simulink model "rlflight"  (R2022b)
settings: Solver=ode45  StartTime=0.0  StopTime=inf  RelTol=1e-3  EnableMultiTasking=on
libraries: instrumentlib x6, rllib x2
settings Model: PacingRate=10  Creator=The MathWorks, Inc.  LastModifiedBy=zzh
settings SolverCC: AlgebraicLoopSolver=TrustRegion
settings DataIOCC: LimitDataPoints=on  SaveFormat=Array  SignalLoggingName=logsOut
settings OptimizationCC: ExpressionDepthLimit=2147483647  InitFltsAndDblsToZero=on  LifeSpan=inf
settings DebuggingCC: SaveWithParameterizedLinksMsg=none  UnderspecifiedInitializationDetection=Classic  MergeDetectMultiDrivingBlocksExec=none  SignalResolutionControl=TryResolveAllWithWarning  MultiTaskDSMMsg=warning  FcnCallInpInsideContextMsg=warning  UnconnectedInputMsg=warning  UnconnectedOutputMsg=warning  UnconnectedLineMsg=warning  AllowSymbolicDim=off  StateNameClashWarn=warning  SFUnexpectedBacktrackingDiag=warning  SFNoUnconditionalDefaultTransitionDiag=warning  SFExecutionAtInitializationDiag=none  SFMachineParentedDataDiag=warning  ArithmeticOperatorsInVariantConditions=warning
settings HardwareCC: ProdBitPerPointer=32  ProdBitPerSizeT=32  ProdBitPerPtrDiffT=32  ProdLargestAtomicFloat=None  ProdIntDivRoundTo=Undefined  ProdEndianess=Unspecified  ProdWordSize=32  ProdHWDeviceType=Specified
settings ModelReferenceCC: EnableRefExpFcnMdlSchedulingChecks=on  PropagateSignalLabelsOutOfModel=off
settings SFSimCC: SimUseLocalCustomCode=off  CustomCodeUndefinedFunction=UseInterfaceOnly
settings RTWCC: RTWUseLocalCustomCode=off  DLArmComputeVersion=19.05
settings CodeAppCC: StateflowObjectComments=on
settings GRTTargetCC: TargetFcnLib=ansi_tfl_tmw.mat  TargetLangStandard=C89/C90 (ANSI)  CombineOutputUpdateFcns=off  GRTInterface=on
settings ConfigComp: CovMetricSettings=dw  CovSaveCumulativeToWorkspaceVar=on  CovSaveSingleToWorkspaceVar=on  CovExternalEMLEnable=off

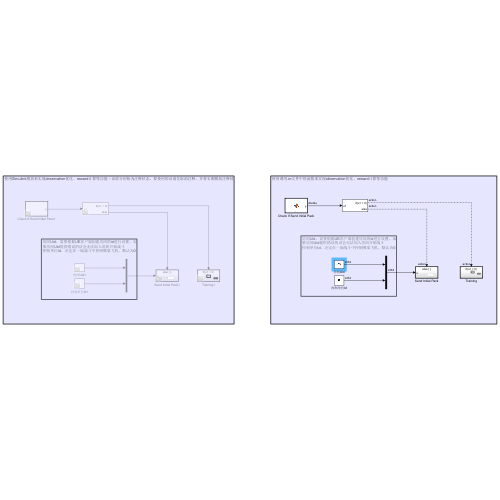
[thumbnail: Simulink's stored preview of the top-level diagram]
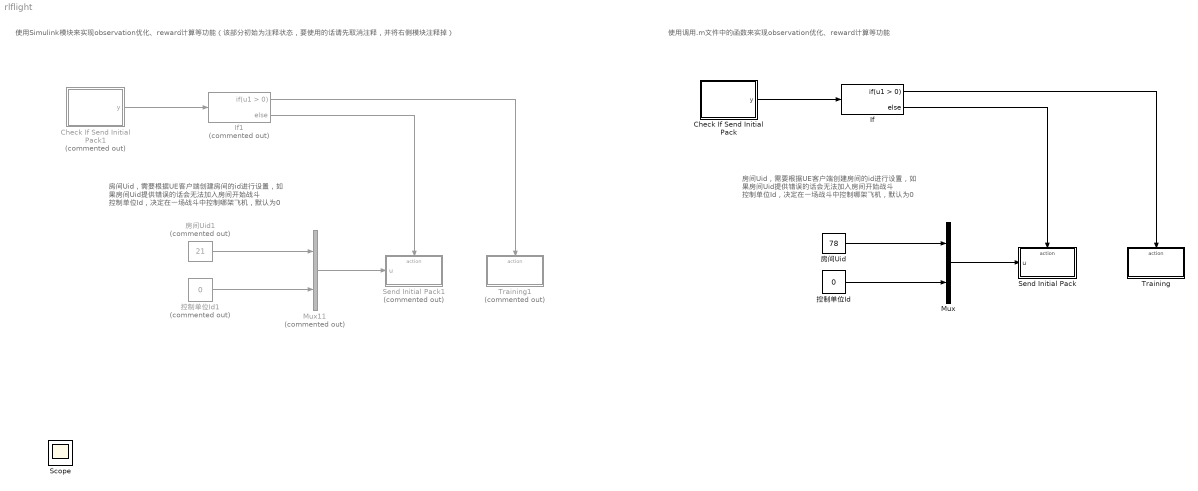
== system rlflight ==
  note: 使用调用.m文件中的函数来实现observation优化、reward计算等功能
  note: 使用Simulink模块来实现observation优化、reward计算等功能（该部分初始为注释状态，要使用的话请先取消注释，并将右侧模块注释掉）
  note: 房间Uid，需要根据UE客户端创建房间的id进行设置，如
      | 果房间Uid提供错误的话会无法加入房间开始战斗
      | 控制单位Id，决定在一场战斗中控制哪架飞机，默认为0
  note: 房间Uid，需要根据UE客户端创建房间的id进行设置，如
      | 果房间Uid提供错误的话会无法加入房间开始战斗
      | 控制单位Id，决定在一场战斗中控制哪架飞机，默认为0
  Check If Send Initial Pack : MATLAB Function  TreatAsAtomicUnit=on
  Check If Send Initial Pack1 : MATLAB Function  Commented=on  TreatAsAtomicUnit=on
  If : If
  If1 : If  Commented=on
  Mux : Mux  Inputs=2
  Mux11 : Mux  Commented=on  Inputs=2
  Send Initial Pack : Subsystem  TreatAsAtomicUnit=on
  Send Initial Pack1 : Subsystem  Commented=on  TreatAsAtomicUnit=on
  Training : Subsystem  TreatAsAtomicUnit=on
  Training1 : Subsystem  Commented=on  TreatAsAtomicUnit=on
  房间Uid : Constant  Value=78  OutDataTypeStr=int32
  房间Uid1 : Constant  Commented=on  Value=21  OutDataTypeStr=int32
  控制单位Id : Constant  Value=0  OutDataTypeStr=int32
  控制单位Id1 : Constant  Commented=on  Value=0  OutDataTypeStr=int32
  Scope : Scope
  wires:
  房间Uid/1 -> Mux/1
  控制单位Id/1 -> Mux/2
  Check If Send Initial Pack/1(y) -> If/1
  Mux/1 -> Send Initial Pack/1(u)
  If/2 -> Send Initial Pack/Action
  If/1 -> Training/Action
  控制单位Id1/1 -> Mux11/2
  Mux11/1 -> Send Initial Pack1/1(u)
  Check If Send Initial Pack1/1(y) -> If1/1
  房间Uid1/1 -> Mux11/1
  If1/2 -> Send Initial Pack1/Action
  If1/1 -> Training1/Action

== system rlflight/Send Initial Pack ==
  u : Inport
  Action Port : ActionPort  ActionPortLabel=else
  TCP发送初始信息 : instrumentlib/TCP//IP Send  Priority=1  Host=127.0.0.1  Port=8080  ByteOrder=little-endian  EnableBlockingMode=on  Timeout=5  TransferDelay=on  SimulateUsing=Interpreted execution
  wires:
  u/1 -> TCP发送初始信息/1

== system rlflight/Send Initial Pack1 ==
  u : Inport
  Action Port : ActionPort  ActionPortLabel=else
  TCP发送初始信息 : instrumentlib/TCP//IP Send  Priority=1  Host=127.0.0.1  Port=8080  ByteOrder=little-endian  EnableBlockingMode=on  Timeout=5  TransferDelay=on  SimulateUsing=Interpreted execution
  wires:
  u/1 -> TCP发送初始信息/1

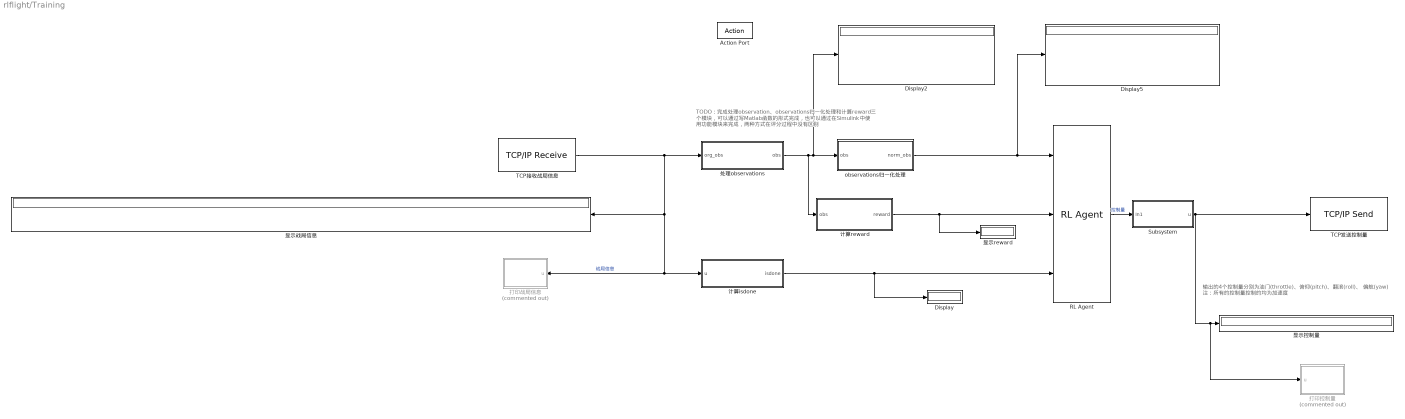
== system rlflight/Training ==
  note: 输出的4个控制量分别为油门(throttle)、俯仰(pitch)、翻滚(roll)、
      | 偏航(yaw)
      | 注：所有的控制量控制的均为加速度
  note: TODO：完成处理observation、observations归一化处理和计算reward三
      | 个模块，可以通过写Matlab函数的形式完成，也可以通过在Simulink中使
      | 用功能模块来完成，两种方式在评分过程中没有区别
  Action Port : ActionPort  ActionPortLabel=if(u1 > 0)
  Display : Display
  Display2 : Display
  Display5 : Display
  RL Agent : rllib/RL Agent  Agent=agent  ExternalActionAsInput=off  ProvideLastAction=off  ProvideCumRwd=off  TreatAsDirectFeedthrough=on  UseStrictObservationDataTypes=off
  Subsystem : Subsystem
  TCP发送控制量 : instrumentlib/TCP//IP Send  Priority=3  Host=127.0.0.1  Port=8080  ByteOrder=little-endian  EnableBlockingMode=on  Timeout=20  TransferDelay=off  SimulateUsing=Interpreted execution
  TCP接收战局信息 : instrumentlib/TCP//IP Receive  Priority=2  Host=127.0.0.1  Port=8080  DataSize=[ 1, 27 ]  DataType=double  ASCIIFormatting=%f  Terminator=LF  CustomTerminator=10  ByteOrder=little-endian  EnableBlockingMode=on  Timeout=20  SampleTime=-1  SimulateUsing=Interpreted execution
  observations归一化处理 : MATLAB Function  TreatAsAtomicUnit=on
  处理observations : MATLAB Function  TreatAsAtomicUnit=on
  打印战局信息 : MATLAB Function  Commented=on  TreatAsAtomicUnit=on
  打印控制量 : MATLAB Function  Commented=on  TreatAsAtomicUnit=on
  显示reward : Display
  显示战局信息 : Display
  显示控制量 : Display
  计算isdone : MATLAB Function  TreatAsAtomicUnit=on
  计算reward : MATLAB Function  TreatAsAtomicUnit=on
  wires:
  计算reward/1(reward) -> 显示reward/1, RL Agent/2
  计算isdone/1(isdone) -> Display/1, RL Agent/3
  TCP接收战局信息/1 -> 打印战局信息/1(u), 计算isdone/1(u), 显示战局信息/1, 处理observations/1(org_obs)  "战局信息"
  observations归一化处理/1(norm_obs) -> Display5/1, RL Agent/1
  处理observations/1(obs) -> 计算reward/1(obs), Display2/1, observations归一化处理/1(obs)
  RL Agent/1 -> Subsystem/1(In1)  "控制量"
  Subsystem/1(u) -> 打印控制量/1(u), 显示控制量/1, TCP发送控制量/1

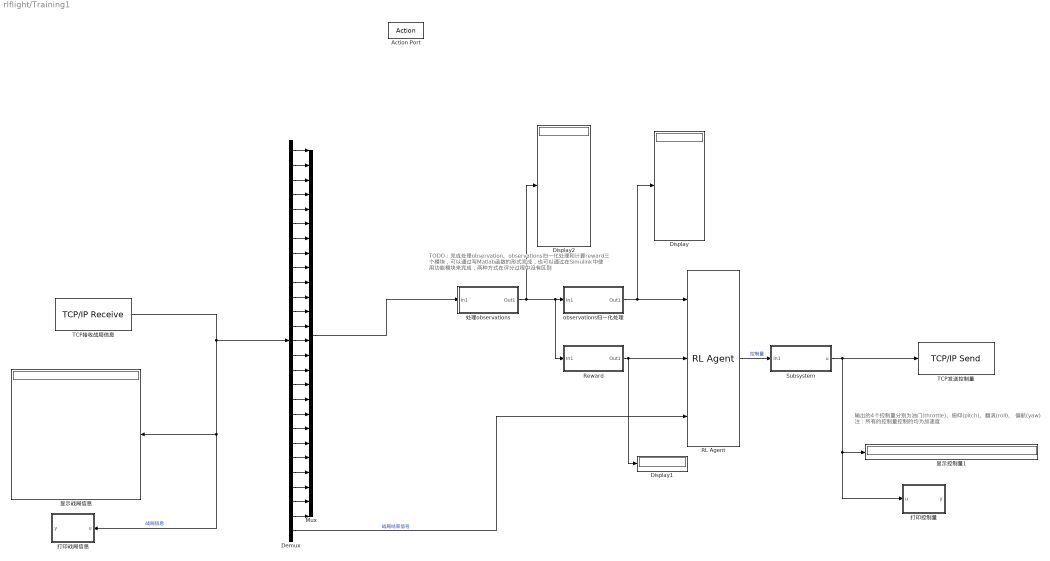
== system rlflight/Training1 ==
  note: 输出的4个控制量分别为油门(throttle)、俯仰(pitch)、翻滚(roll)、
      | 偏航(yaw)
      | 注：所有的控制量控制的均为加速度
  note: TODO：完成处理observation、observations归一化处理和计算reward三
      | 个模块，可以通过写Matlab函数的形式完成，也可以通过在Simulink中使
      | 用功能模块来完成，两种方式在评分过程中没有区别
  Action Port : ActionPort  ActionPortLabel=if(u1 > 0)
  Demux : Demux  Outputs=27
  Display : Display
  Display1 : Display
  Display2 : Display
  Mux : Mux  Inputs=26
  RL Agent : rllib/RL Agent  Agent=agent  ExternalActionAsInput=off  ProvideLastAction=off  ProvideCumRwd=off  TreatAsDirectFeedthrough=on  UseStrictObservationDataTypes=off
  Reward : Subsystem
  Subsystem : Subsystem
  TCP发送控制量 : instrumentlib/TCP//IP Send  Priority=3  Host=127.0.0.1  Port=8080  ByteOrder=little-endian  EnableBlockingMode=on  Timeout=30  TransferDelay=off  SimulateUsing=Interpreted execution
  TCP接收战局信息 : instrumentlib/TCP//IP Receive  Priority=2  Host=127.0.0.1  Port=8080  DataSize=[ 1, 27 ]  DataType=double  ASCIIFormatting=%f  Terminator=LF  CustomTerminator=10  ByteOrder=little-endian  EnableBlockingMode=on  Timeout=30  SampleTime=-1  SimulateUsing=Interpreted execution
  observations归一化处理 : Subsystem
  处理observations : Subsystem
  打印战局信息 : MATLAB Function  TreatAsAtomicUnit=on
  打印控制量 : MATLAB Function  TreatAsAtomicUnit=on
  显示战局信息 : Display
  显示控制量1 : Display
  wires:
  TCP接收战局信息/1 -> 打印战局信息/1(u), 显示战局信息/1, Demux/1  "战局信息"
  RL Agent/1 -> Subsystem/1(In1)  "控制量"
  Demux/27 -> RL Agent/3  "战局结束信号"
  observations归一化处理/1(Out1) -> Display/1, RL Agent/1
  处理observations/1(Out1) -> Display2/1, Reward/1(In1), observations归一化处理/1(In1)
  Demux/13 -> Mux/13
  Demux/12 -> Mux/12
  Demux/11 -> Mux/11
  Demux/10 -> Mux/10
  Demux/9 -> Mux/9
  Demux/8 -> Mux/8
  Demux/7 -> Mux/7
  Demux/6 -> Mux/6
  Demux/5 -> Mux/5
  Demux/4 -> Mux/4
  Demux/3 -> Mux/3
  Demux/2 -> Mux/2
  Demux/1 -> Mux/1
  Demux/14 -> Mux/14
  Demux/15 -> Mux/15
  Demux/16 -> Mux/16
  Demux/17 -> Mux/17
  Demux/18 -> Mux/18
  Demux/19 -> Mux/19
  Demux/20 -> Mux/20
  Demux/21 -> Mux/21
  Demux/22 -> Mux/22
  Demux/23 -> Mux/23
  Demux/24 -> Mux/24
  Demux/25 -> Mux/25
  Demux/26 -> Mux/26
  Mux/1 -> 处理observations/1(In1)
  Reward/1(Out1) -> Display1/1, RL Agent/2
  Subsystem/1(u) -> TCP发送控制量/1, 打印控制量/1(u), 显示控制量1/1

== system rlflight/Training/Subsystem ==
  In1 : Inport
  Constant : Constant  Value=0
  Demux : Demux  Outputs=3
  Mux : Mux
  u : Outport
  wires:
  In1/1 -> Demux/1
  Mux/1 -> u/1
  Constant/1 -> Mux/3
  Demux/1 -> Mux/1
  Demux/2 -> Mux/2
  Demux/3 -> Mux/4

== system rlflight/Training1/Reward ==
  In1 : Inport
  Add1 : Sum  Inputs=+++
  Demux : Demux  Outputs=11
  Magnitude Squared : Math  Operator=square
  Magnitude Squared1 : Math  Operator=square
  Magnitude Squared2 : Math  Operator=square
  S-Function Builder : S-Function  FunctionName=TrackReward  SFunctionModules=TrackReward_wrapper.c  SFunctionDeploymentMode=off  EnableBusSupport=off  mask(S-Function Builder){}
      mask help: Simulink:masks:SFunctionBuilder_MD
      mask init:
      | val = [[.9  0.75 0.75 1 1 .9 .9 1]',[1 1 0.75 0.75 .9 .9 1 .9]'];try , sys = get_param(gcb,'SfunBuilderFcnName');if isempty(sys), sys = get_param(gcb,'FunctionName'); end,catch, sys = get_param(gcb,'FunctionName'); end
      settings: CopyFcn=set_param(gcbh,'LinkStatus','none')  OpenFcn=sfunctionwizard(gcbh)
      mask Display:
      | plot(val(:,1),val(:,2))
      | disp(sys)
      | port_label('input',1,'r')
      | port_label('input',2,'pitch_diff')
      | port_label('input',3,'yaw_diff')
      | port_label('input',4,'enemy_pitch_diff')
      | port_label('input',5,'enemy_yaw_diff')
      | port_label('input',6,'enemy_hp')
      | port_label('output',1,'reward')
  Sqrt : Sqrt
  Out1 : Outport
  wires:
  In1/1 -> Demux/1
  Magnitude Squared/1 -> Add1/1
  Magnitude Squared1/1 -> Add1/2
  Magnitude Squared2/1 -> Add1/3
  Add1/1 -> Sqrt/1
  Sqrt/1 -> S-Function Builder/1
  S-Function Builder/1 -> Out1/1
  Demux/1 -> Magnitude Squared/1
  Demux/2 -> Magnitude Squared1/1
  Demux/3 -> Magnitude Squared2/1
  Demux/7 -> S-Function Builder/2
  Demux/8 -> S-Function Builder/3
  Demux/9 -> S-Function Builder/4
  Demux/10 -> S-Function Builder/5
  Demux/11 -> S-Function Builder/6

== system rlflight/Training1/Subsystem ==
  In1 : Inport
  Constant : Constant  Value=0
  Constant2 : Constant  Value=0
  Demux : Demux  Outputs=2
  Mux : Mux
  u : Outport
  wires:
  In1/1 -> Demux/1
  Mux/1 -> u/1
  Constant/1 -> Mux/3
  Constant2/1 -> Mux/1
  Demux/2 -> Mux/4
  Demux/1 -> Mux/2

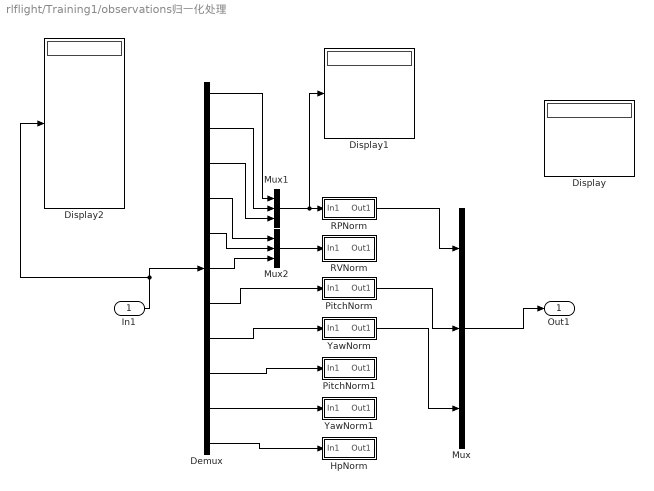
== system rlflight/Training1/observations归一化处理 ==
  In1 : Inport
  Demux : Demux  Outputs=11
  Display : Display
  Display1 : Display
  Display2 : Display
  HpNorm : Subsystem
  Mux : Mux  Inputs=3
  Mux1 : Mux  Inputs=3
  Mux2 : Mux  Inputs=3
  PitchNorm : Subsystem
  PitchNorm1 : Subsystem
  RPNorm : Subsystem
  RVNorm : Subsystem
  YawNorm : Subsystem
  YawNorm1 : Subsystem
  Out1 : Outport
  wires:
  In1/1 -> Display2/1, Demux/1
  Mux/1 -> Out1/1
  RPNorm/1(Out1) -> Mux/1
  PitchNorm/1(Out1) -> Mux/2
  Demux/10 -> YawNorm1/1(In1)
  Demux/9 -> PitchNorm1/1(In1)
  Demux/8 -> YawNorm/1(In1)
  Demux/7 -> PitchNorm/1(In1)
  Mux1/1 -> Display1/1, RPNorm/1(In1)
  Mux2/1 -> RVNorm/1(In1)
  Demux/1 -> Mux1/1
  Demux/2 -> Mux1/2
  Demux/3 -> Mux1/3
  Demux/4 -> Mux2/1
  Demux/5 -> Mux2/2
  Demux/6 -> Mux2/3
  YawNorm/1(Out1) -> Mux/3
  Demux/11 -> HpNorm/1(In1)

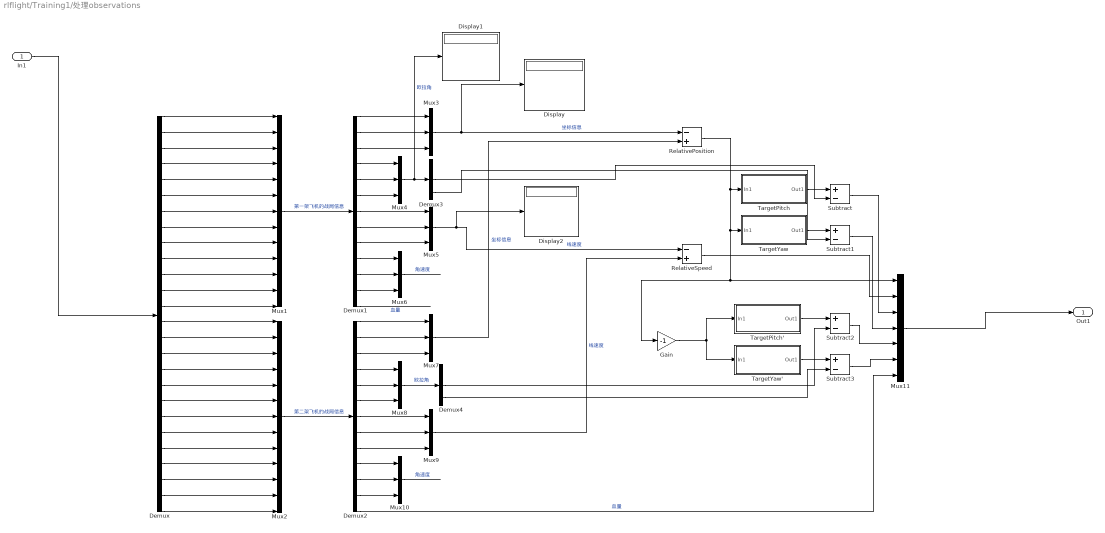
== system rlflight/Training1/处理observations ==
  In1 : Inport
  Demux : Demux  Outputs=26
  Demux1 : Demux  Outputs=13
  Demux2 : Demux  Outputs=13
  Demux3 : Demux  Outputs=3
  Demux4 : Demux  Outputs=3
  Display : Display
  Display1 : Display
  Display2 : Display
  Gain : Gain  Gain=-1
  Mux1 : Mux  Inputs=13
  Mux{3..10} (8 alike) : Mux  Inputs=3
  Mux11 : Mux  Inputs=7
  Mux2 : Mux  Inputs=13
  RelativePosition : Sum  Inputs=-+
  RelativeSpeed : Sum  Inputs=-+
  Subtract{,1..3} (4 alike) : Sum  Inputs=+-
  TargetPitch : Subsystem
  TargetPitch' : Subsystem
  TargetYaw : Subsystem
  TargetYaw' : Subsystem
  Out1 : Outport
  wires:
  In1/1 -> Demux/1
  Mux10/1 -> ?  "角速度"
  Demux/3 -> Mux1/3
  Demux/4 -> Mux1/4
  Demux1/2 -> Mux3/2
  Mux9/1 -> RelativeSpeed/2  "线速度"
  Demux/12 -> Mux1/12
  Demux/1 -> Mux1/1
  Demux1/8 -> Mux5/2
  Demux1/12 -> Mux6/3
  Demux1/4 -> Mux4/1
  Demux/9 -> Mux1/9
  Demux1/6 -> Mux4/3
  Mux8/1 -> Demux4/1  "欧拉角"
  Demux/25 -> Mux2/12
  Demux2/9 -> Mux9/3
  Demux2/13 -> Mux11/7  "血量"
  Demux2/4 -> Mux8/1
  Demux/7 -> Mux1/7
  Mux5/1 -> Display2/1, RelativeSpeed/1  "线速度"
  Demux2/11 -> Mux10/2
  Mux4/1 -> Display1/1, Demux3/1  "欧拉角"
  Demux2/2 -> Mux7/2
  Demux2/8 -> Mux9/2
  Demux/22 -> Mux2/9
  Demux/20 -> Mux2/7
  Demux2/12 -> Mux10/3
  Demux/6 -> Mux1/6
  Demux/26 -> Mux2/13
  Demux1/9 -> Mux5/3
  Demux/11 -> Mux1/11
  Demux2/5 -> Mux8/2
  Demux1/1 -> Mux3/1
  Demux1/10 -> Mux6/1
  Demux/14 -> Mux2/1
  Demux2/1 -> Mux7/1
  Demux/5 -> Mux1/5
  Demux1/7 -> Mux5/1
  Demux/24 -> Mux2/11
  Mux6/1 -> ?  "角速度"
  Demux/18 -> Mux2/5
  Mux1/1 -> Demux1/1  "第一架飞机的战局信息"
  Demux/10 -> Mux1/10
  Demux/13 -> Mux1/13
  Demux2/3 -> Mux7/3
  Demux/8 -> Mux1/8
  Mux2/1 -> Demux2/1  "第二架飞机的战局信息"
  Demux2/10 -> Mux10/1
  Demux/16 -> Mux2/3
  Demux2/6 -> Mux8/3
  Demux/2 -> Mux1/2
  Demux/19 -> Mux2/6
  Demux1/5 -> Mux4/2
  Demux/23 -> Mux2/10
  Demux/21 -> Mux2/8
  Demux1/3 -> Mux3/3
  Demux/17 -> Mux2/4
  Demux1/11 -> Mux6/2
  Demux1/13 -> ?  "血量"
  Demux/15 -> Mux2/2
  Demux2/7 -> Mux9/1
  Subtract3/1 -> Mux11/6
  RelativeSpeed/1 -> Mux11/2
  Mux11/1 -> Out1/1
  Subtract/1 -> Mux11/3
  Mux3/1 -> Display/1, RelativePosition/1  "坐标信息"
  TargetYaw/1(Out1) -> Subtract1/1
  TargetPitch/1(Out1) -> Subtract/1
  Subtract2/1 -> Mux11/5
  TargetPitch'/1(Out1) -> Subtract2/1
  RelativePosition/1 -> TargetPitch/1(In1), TargetYaw/1(In1), Gain/1, Mux11/1
  Subtract1/1 -> Mux11/4
  TargetYaw'/1(Out1) -> Subtract3/1
  Mux7/1 -> RelativePosition/2  "坐标信息"
  Demux3/2 -> Subtract/2
  Demux3/3 -> Subtract1/2
  Demux4/2 -> Subtract2/2
  Demux4/3 -> Subtract3/2
  Gain/1 -> TargetYaw'/1(In1), TargetPitch'/1(In1)

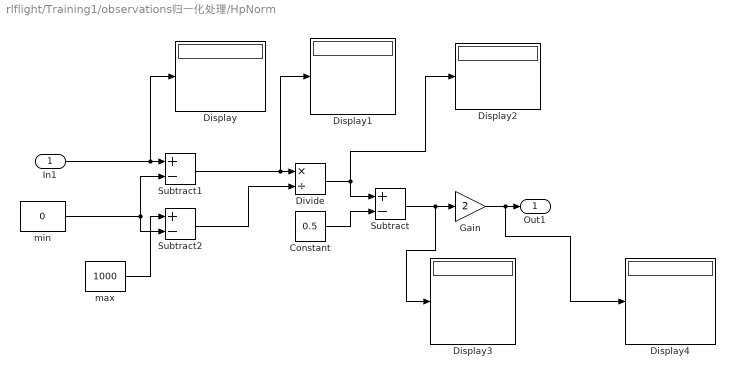
== system rlflight/Training1/observations归一化处理/HpNorm ==
  In1 : Inport
  Constant : Constant  Value=0.5
  Display{,1..4} (5 alike) : Display
  Divide : Product  Inputs=*/
  Gain : Gain  Gain=2
  Subtract : Sum  Inputs=+-
  Subtract1 : Sum  Inputs=+-
  Subtract2 : Sum  Inputs=+-
  max : Constant  Value=1000
  min : Constant  Value=0
  Out1 : Outport
  wires:
  Gain/1 -> Display4/1, Out1/1
  Divide/1 -> Display2/1, Subtract/1
  Constant/1 -> Subtract/2
  Subtract/1 -> Display3/1, Gain/1
  In1/1 -> Display/1, Subtract1/1
  min/1 -> Subtract2/2, Subtract1/2
  Subtract1/1 -> Display1/1, Divide/1
  Subtract2/1 -> Divide/2
  max/1 -> Subtract2/1

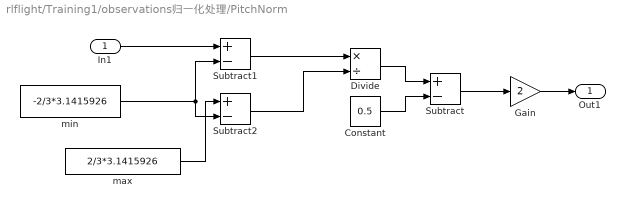
== system rlflight/Training1/observations归一化处理/PitchNorm ==
  In1 : Inport
  Constant : Constant  Value=0.5
  Divide : Product  Inputs=*/
  Gain : Gain  Gain=2
  Subtract : Sum  Inputs=+-
  Subtract1 : Sum  Inputs=+-
  Subtract2 : Sum  Inputs=+-
  max : Constant  Value=2/3*3.1415926
  min : Constant  Value=-2/3*3.1415926
  Out1 : Outport
  wires:
  Gain/1 -> Out1/1
  Divide/1 -> Subtract/1
  Constant/1 -> Subtract/2
  Subtract/1 -> Gain/1
  In1/1 -> Subtract1/1
  min/1 -> Subtract1/2, Subtract2/2
  Subtract1/1 -> Divide/1
  Subtract2/1 -> Divide/2
  max/1 -> Subtract2/1

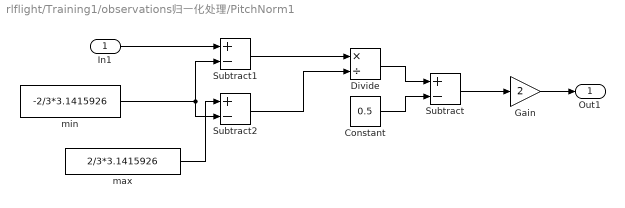
== system rlflight/Training1/observations归一化处理/PitchNorm1 ==
  In1 : Inport
  Constant : Constant  Value=0.5
  Divide : Product  Inputs=*/
  Gain : Gain  Gain=2
  Subtract : Sum  Inputs=+-
  Subtract1 : Sum  Inputs=+-
  Subtract2 : Sum  Inputs=+-
  max : Constant  Value=2/3*3.1415926
  min : Constant  Value=-2/3*3.1415926
  Out1 : Outport
  wires:
  Gain/1 -> Out1/1
  Divide/1 -> Subtract/1
  Constant/1 -> Subtract/2
  Subtract/1 -> Gain/1
  In1/1 -> Subtract1/1
  min/1 -> Subtract1/2, Subtract2/2
  Subtract1/1 -> Divide/1
  Subtract2/1 -> Divide/2
  max/1 -> Subtract2/1

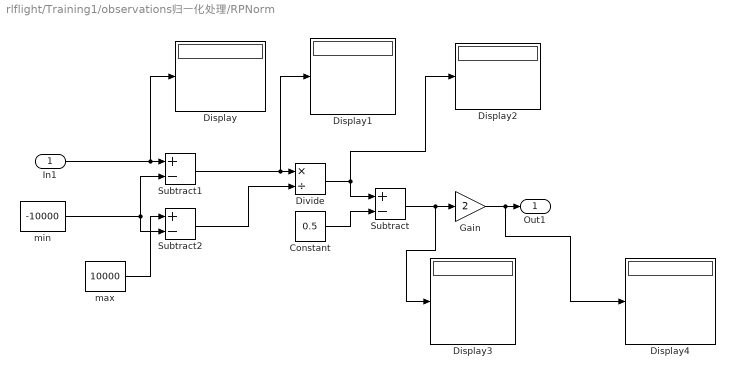
== system rlflight/Training1/observations归一化处理/RPNorm ==
  In1 : Inport
  Constant : Constant  Value=0.5
  Display{,1..4} (5 alike) : Display
  Divide : Product  Inputs=*/
  Gain : Gain  Gain=2
  Subtract : Sum  Inputs=+-
  Subtract1 : Sum  Inputs=+-
  Subtract2 : Sum  Inputs=+-
  max : Constant  Value=10000
  min : Constant  Value=-10000
  Out1 : Outport
  wires:
  Gain/1 -> Display4/1, Out1/1
  Divide/1 -> Display2/1, Subtract/1
  Constant/1 -> Subtract/2
  Subtract/1 -> Display3/1, Gain/1
  In1/1 -> Display/1, Subtract1/1
  min/1 -> Subtract2/2, Subtract1/2
  Subtract1/1 -> Display1/1, Divide/1
  Subtract2/1 -> Divide/2
  max/1 -> Subtract2/1

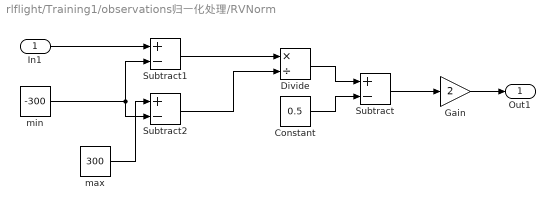
== system rlflight/Training1/observations归一化处理/RVNorm ==
  In1 : Inport
  Constant : Constant  Value=0.5
  Divide : Product  Inputs=*/
  Gain : Gain  Gain=2
  Subtract : Sum  Inputs=+-
  Subtract1 : Sum  Inputs=+-
  Subtract2 : Sum  Inputs=+-
  max : Constant  Value=300
  min : Constant  Value=-300
  Out1 : Outport
  wires:
  Gain/1 -> Out1/1
  Divide/1 -> Subtract/1
  Constant/1 -> Subtract/2
  Subtract/1 -> Gain/1
  In1/1 -> Subtract1/1
  min/1 -> Subtract2/2, Subtract1/2
  Subtract1/1 -> Divide/1
  Subtract2/1 -> Divide/2
  max/1 -> Subtract2/1

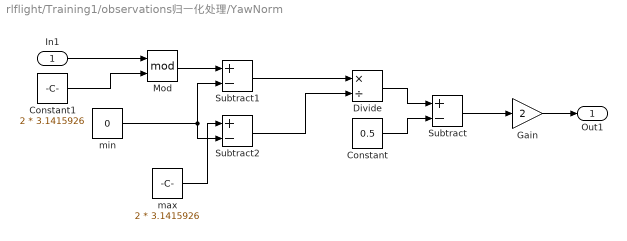
== system rlflight/Training1/observations归一化处理/YawNorm ==
  In1 : Inport
  Constant : Constant  Value=0.5
  Constant1 : Constant  Value=2 * 3.1415926
  Divide : Product  Inputs=*/
  Gain : Gain  Gain=2
  Mod : Math  Operator=mod
  Subtract : Sum  Inputs=+-
  Subtract1 : Sum  Inputs=+-
  Subtract2 : Sum  Inputs=+-
  max : Constant  Value=2 * 3.1415926
  min : Constant  Value=0
  Out1 : Outport
  wires:
  Gain/1 -> Out1/1
  Divide/1 -> Subtract/1
  Constant/1 -> Subtract/2
  Subtract/1 -> Gain/1
  min/1 -> Subtract2/2, Subtract1/2
  Subtract1/1 -> Divide/1
  Subtract2/1 -> Divide/2
  max/1 -> Subtract2/1
  Mod/1 -> Subtract1/1
  In1/1 -> Mod/1
  Constant1/1 -> Mod/2

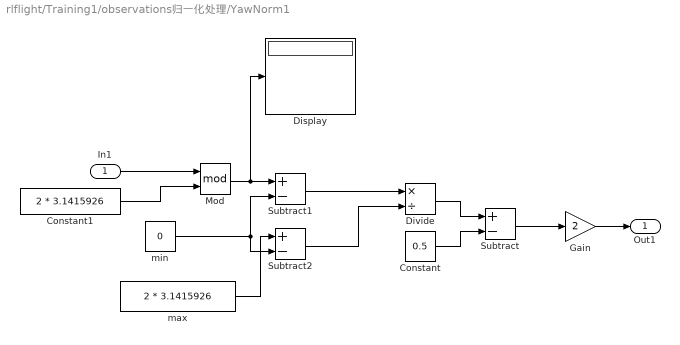
== system rlflight/Training1/observations归一化处理/YawNorm1 ==
  In1 : Inport
  Constant : Constant  Value=0.5
  Constant1 : Constant  Value=2 * 3.1415926
  Display : Display
  Divide : Product  Inputs=*/
  Gain : Gain  Gain=2
  Mod : Math  Operator=mod
  Subtract : Sum  Inputs=+-
  Subtract1 : Sum  Inputs=+-
  Subtract2 : Sum  Inputs=+-
  max : Constant  Value=2 * 3.1415926
  min : Constant  Value=0
  Out1 : Outport
  wires:
  Gain/1 -> Out1/1
  Divide/1 -> Subtract/1
  Constant/1 -> Subtract/2
  Subtract/1 -> Gain/1
  min/1 -> Subtract2/2, Subtract1/2
  Subtract1/1 -> Divide/1
  Subtract2/1 -> Divide/2
  max/1 -> Subtract2/1
  Mod/1 -> Display/1, Subtract1/1
  In1/1 -> Mod/1
  Constant1/1 -> Mod/2

== system rlflight/Training1/处理observations/TargetPitch ==
  In1 : Inport
  Add : Sum
  Atan : Trigonometry  Operator=atan
  Demux : Demux  Outputs=3
  Divide : Product  Inputs=/*
  Sqrt : Sqrt
  Square : Math  Operator=square
  Square1 : Math  Operator=square
  Out1 : Outport
  wires:
  In1/1 -> Demux/1
  Atan/1 -> Out1/1
  Demux/3 -> Divide/2
  Sqrt/1 -> Divide/1
  Divide/1 -> Atan/1
  Square/1 -> Add/1
  Add/1 -> Sqrt/1
  Demux/1 -> Square/1
  Square1/1 -> Add/2
  Demux/2 -> Square1/1

== system rlflight/Training1/处理observations/TargetPitch' ==
  In1 : Inport
  Add : Sum
  Atan : Trigonometry  Operator=atan
  Demux : Demux  Outputs=3
  Divide : Product  Inputs=/*
  Sqrt : Sqrt
  Square : Math  Operator=square
  Square1 : Math  Operator=square
  Out1 : Outport
  wires:
  In1/1 -> Demux/1
  Atan/1 -> Out1/1
  Demux/3 -> Divide/2
  Sqrt/1 -> Divide/1
  Divide/1 -> Atan/1
  Square/1 -> Add/1
  Add/1 -> Sqrt/1
  Demux/1 -> Square/1
  Square1/1 -> Add/2
  Demux/2 -> Square1/1

== system rlflight/Training1/处理observations/TargetYaw ==
  In1 : Inport
  Add : Sum
  Atan : Trigonometry  Operator=atan
  Constant : Constant  Value=3.1415926
  Demux : Demux  Outputs=3
  Divide : Product  Inputs=/*
  Switch : Switch  Criteria=u2 > Threshold  SaturateOnIntegerOverflow=off  InputSameDT=off
  Out1 : Outport
  wires:
  In1/1 -> Demux/1
  Demux/1 -> Divide/1, Switch/2
  Switch/1 -> Out1/1
  Demux/2 -> Divide/2
  Divide/1 -> Atan/1
  Atan/1 -> Switch/1, Add/1
  Add/1 -> Switch/3
  Constant/1 -> Add/2

== system rlflight/Training1/处理observations/TargetYaw' ==
  In1 : Inport
  Add : Sum
  Atan : Trigonometry  Operator=atan
  Constant : Constant  Value=3.1415926
  Demux : Demux  Outputs=3
  Divide : Product  Inputs=/*
  Switch : Switch  Criteria=u2 > Threshold  SaturateOnIntegerOverflow=off  InputSameDT=off
  Out1 : Outport
  wires:
  In1/1 -> Demux/1
  Demux/1 -> Divide/1, Switch/2
  Switch/1 -> Out1/1
  Demux/2 -> Divide/2
  Divide/1 -> Atan/1
  Atan/1 -> Switch/1, Add/1
  Add/1 -> Switch/3
  Constant/1 -> Add/2

== matlab function rlflight/Training1/打印战局信息 ==
  data: u input; y output
function y = fcn(u)
fprintf('position = \n');
disp(u)
fprintf('\n');
y = u;
end

== matlab function rlflight/Check If Send Initial Pack1 ==
  data: y output
function y = fcn()
%判断是否为第一个回合
persistent ifSendInitPack;
if isempty(ifSendInitPack)
    ifSendInitPack = 0;
end
y = ifSendInitPack;
if(ifSendInitPack == 0)
    ifSendInitPack = 1;
end
end

== matlab function rlflight/Training/打印战局信息 ==
  data: u input
function fcn(u)
fprintf('position = \n');
disp(u)
fprintf('\n');
end

== matlab function rlflight/Training/打印控制量 ==
  data: u input
function fcn(u)
fprintf('action = \n');
disp(u)
fprintf('-----------\n');
end

== matlab function rlflight/Training/计算isdone ==
  data: u input; isdone output
function isdone = fcn(u)
isdone = u(27);
end

== matlab function rlflight/Training/计算reward ==
  data: obs input; reward output
function reward = fcn(obs)

persistent pre_obs;
if isempty(pre_obs)
    pre_obs = obs;
end

reward = get_my_reward(obs, pre_obs);

pre_obs = obs;
end

== matlab function rlflight/Training/处理observations ==
  data: org_obs input; obs output
function obs = fcn(org_obs)
    obs = get_my_obs(org_obs);
end

== matlab function rlflight/Training/observations归一化处理 ==
  data: obs input; norm_obs output
function norm_obs = fcn(obs)
norm_obs = normalize_my_obs(obs);
end

== matlab function rlflight/Check If Send Initial Pack ==
  data: y output
function y = fcn()
%判断是否为第一个回合
persistent ifSendInitPack;
if isempty(ifSendInitPack)
    ifSendInitPack = 0;
end
y = ifSendInitPack;
if(ifSendInitPack == 0)
    ifSendInitPack = 1;
end
end

== matlab function rlflight/Training1/打印控制量 ==
  data: u input; y output
function y = fcn(u)
fprintf('action = \n');
disp(u)
fprintf('-----------\n');
y = u;
end
